simulink model "OptimizePID"  (R2020a)
settings: Solver=VariableStepAuto  StartTime=0.0  StopTime=10  RelTol=1e-4
undefined symbols (not defined in the file or in its folder): k
settings Model: Creator=aslam  LastModifiedBy=aslam
settings SolverCC: MaxConsecutiveMinStep=2
settings DataIOCC: ReturnWorkspaceOutputs=off

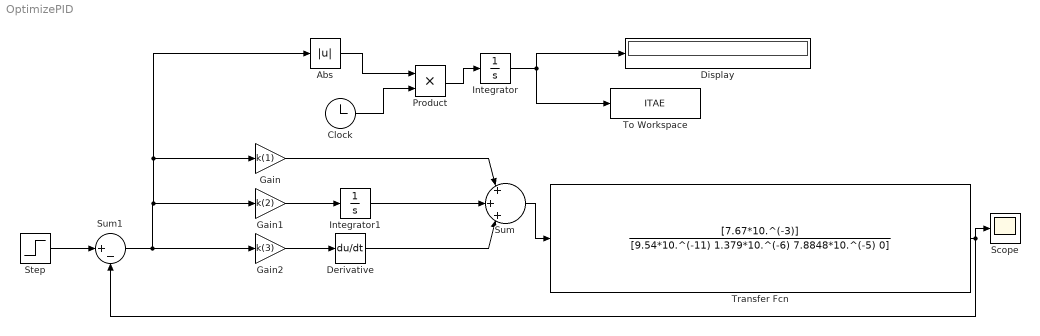
== system OptimizePID ==
  Abs : Abs
  Clock : Clock
  Derivative : Derivative
  Display : Display
      settings: Format=decimal (Stored Integer)
  Gain : Gain  Gain=k(1)
  Gain1 : Gain  Gain=k(2)
  Gain2 : Gain  Gain=k(3)
  Integrator : Integrator
  Integrator1 : Integrator
  Product : Product
  Scope : Scope
  Step : Step  SampleTime=0
  Sum : Sum  Inputs=|+|+|+|
  Sum1 : Sum  Inputs=|+-
  To Workspace : ToWorkspace  VariableName=ITAE  SampleTime=-1
  Transfer Fcn : TransferFcn  Numerator=[7.67*10.^(-3)]  Denominator=[9.54*10.^(-11) 1.379*10.^(-6) 7.8848*10.^(-5) 0]
  wires:
  Gain2/1 -> Derivative/1
  Gain1/1 -> Integrator1/1
  Integrator1/1 -> Sum/2
  Derivative/1 -> Sum/3
  Gain/1 -> Sum/1
  Sum1/1 -> Abs/1, Gain/1, Gain1/1, Gain2/1
  Step/1 -> Sum1/1
  Clock/1 -> Product/2
  Abs/1 -> Product/1
  Product/1 -> Integrator/1
  Sum/1 -> Transfer Fcn/1
  Transfer Fcn/1 -> Scope/1, Sum1/2
  Integrator/1 -> To Workspace/1, Display/1
